simulink model "AFS_Master_Test"  (R2020b)
settings: configuration reference "VLS_Standard_Configuration" (kept outside this file)
settings Model: DataDictionary=AFS_Master_Model.sldd  Creator=mmoufakk  LastModifiedBy=mtarek-a
settings ConfigSetRef: SourceName=VLS_Standard_Configuration

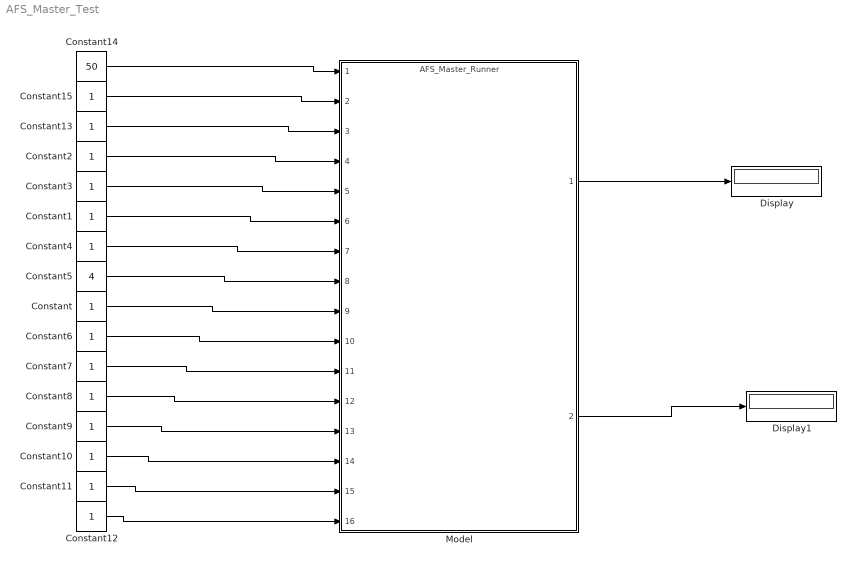
== system AFS_Master_Test ==
  Constant{,1..4,6..13,15} (14 alike) : Constant  OutDataTypeStr=boolean
  Constant14 : Constant  Value=50  OutDataTypeStr=speed_type
  Constant5 : Constant  Value=4  OutDataTypeStr=uint8
  Display : Display
  Display1 : Display
  Model : ModelReference  ModelNameDialog=AFS_Master_Runner.slx  SimulationMode=Normal  ModelReferenceVersion=1.48
  wires:
  Model/1 -> Display/1
  Model/2 -> Display1/1
  Constant14/1 -> Model/1
  Constant15/1 -> Model/2
  Constant13/1 -> Model/3
  Constant2/1 -> Model/4
  Constant3/1 -> Model/5
  Constant1/1 -> Model/6
  Constant4/1 -> Model/7
  Constant5/1 -> Model/8
  Constant/1 -> Model/9
  Constant6/1 -> Model/10
  Constant7/1 -> Model/11
  Constant8/1 -> Model/12
  Constant9/1 -> Model/13
  Constant10/1 -> Model/14
  Constant11/1 -> Model/15
  Constant12/1 -> Model/16
